simulink model "MC_Phase2_Part1_Q4_Sim"  (R2020b)
settings: Solver=VariableStepAuto  StartTime=0.0  StopTime=15  RelTol=1e-3
settings Model: Creator=ASUS  LastModifiedBy=ASUS

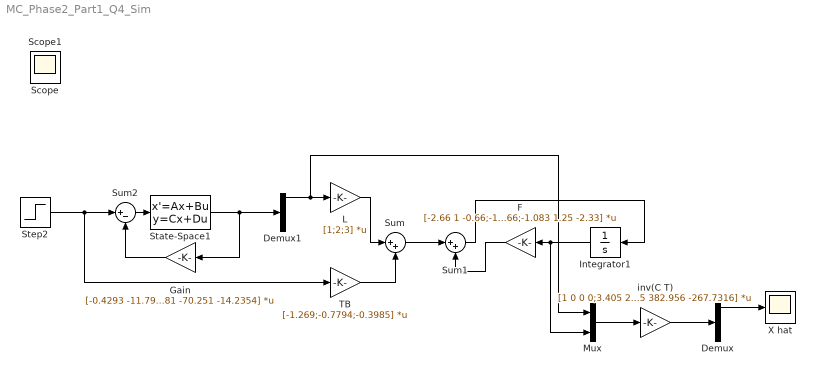
== system MC_Phase2_Part1_Q4_Sim ==
  Demux : Demux
  Demux1 : Demux
  F : Gain  Gain=[-2.66 1 -0.66;-1.33 -1 0.66;-1.083 1.25 -2.33]  Multiplication=Matrix(K*u)
  Gain : Gain  Gain=[-0.4293 -11.7981 -70.251 -14.2354]  Multiplication=Matrix(K*u)
  Integrator1 : Integrator
  L : Gain  Gain=[1;2;3]  Multiplication=Matrix(K*u)
  Mux : Mux  Inputs=2
  State-Space1 : StateSpace  A=[0 1 0 0;0 -2.2626 -0.3963 0.0082;0 0 0 1;0 3.5649 16.0655 -0.3324]  B=[0;0.2263;0;-0.3565]  C=[1 0 0 0;0 1 0 0;0 0 1 0;0 0 0 1]  D=[0;0;0;0]  InitialCondition=0
  Step2 : Step  SampleTime=0
  Sum : Sum  Inputs=|++
  Sum1 : Sum  Inputs=|++
  Sum2 : Sum  Inputs=|+-
  TB : Gain  Gain=[-1.269;-0.7794;-0.3985]  Multiplication=Matrix(K*u)
  X hat : Scope
  inv(C T) : Gain  Gain=[1 0 0 0;3.405 2.6748 -7.8845 6.3356;-68.609 -32.5834 74.0537 -41.0813;-241.3337 -150.8565 382.956 -267.7316]  Multiplication=Matrix(K*u)
  Scope : Scope
  Scope1 : Scope
  wires:
  Step2/1 -> Sum2/1, TB/1
  State-Space1/1 -> Gain/1, Demux1/1
  Demux1/1 -> Mux/1, L/1
  Integrator1/1 -> Mux/2, F/1
  TB/1 -> Sum/2
  L/1 -> Sum/1
  Sum/1 -> Sum1/1
  F/1 -> Sum1/2
  Sum1/1 -> Integrator1/1
  Mux/1 -> inv(C T)/1
  inv(C T)/1 -> Demux/1
  Demux/1 -> X hat/1
  Sum2/1 -> State-Space1/1
  Gain/1 -> Sum2/2
